simulink model "cemilModel"  (R2020b)
settings: Solver=VariableStepAuto  StartTime=0.0  StopTime=10.0  RelTol=1e-3
settings Model: Creator=kuzub  LastModifiedBy=kuzub

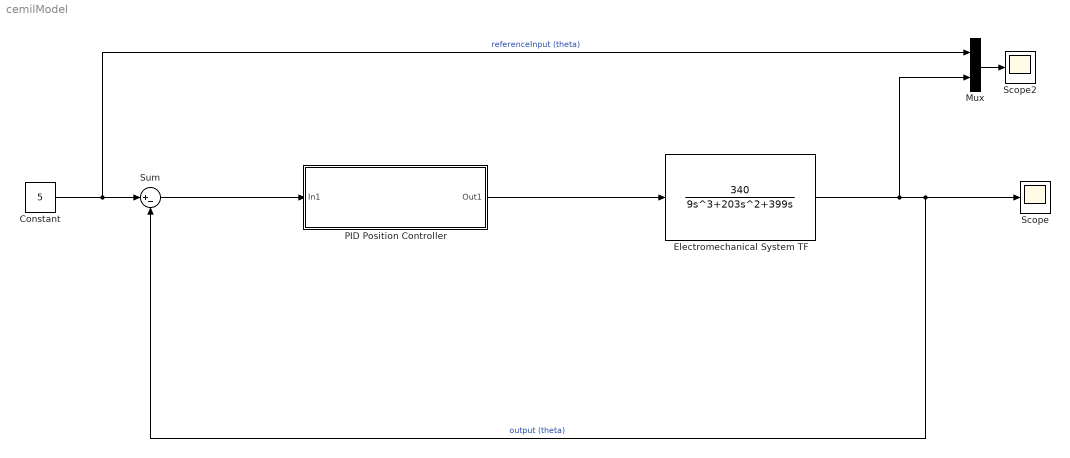
== system cemilModel ==
  Constant : Constant  Value=5
  Electromechanical System TF : TransferFcn  Numerator=[340]  Denominator=[9 203 399 0]
  Mux : Mux  Inputs=2
  PID Position Controller : Subsystem
  Scope : Scope
  Scope2 : Scope
  Sum : Sum  Inputs=|+-
  wires:
  Constant/1 -> Mux/1, Sum/1  "referenceInput (theta)"
  Electromechanical System TF/1 -> Mux/2, Scope/1, Sum/2  "output (theta)"
  Sum/1 -> PID Position Controller/1(In1)
  PID Position Controller/1(Out1) -> Electromechanical System TF/1
  Mux/1 -> Scope2/1

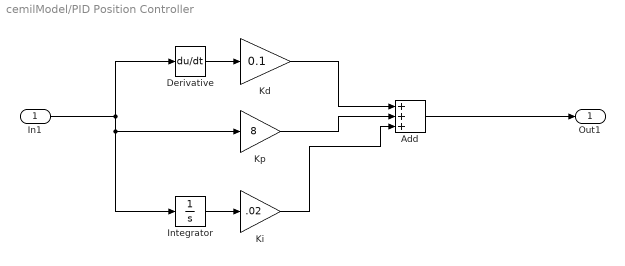
== system cemilModel/PID Position Controller ==
  In1 : Inport
  Add : Sum  Inputs=+++
  Derivative : Derivative
  Integrator : Integrator
  Kd : Gain  Gain=0.1
  Ki : Gain  Gain=.02
  Kp : Gain  Gain=8
  Out1 : Outport
  wires:
  Kd/1 -> Add/1
  In1/1 -> Derivative/1, Integrator/1, Kp/1
  Add/1 -> Out1/1
  Integrator/1 -> Ki/1
  Ki/1 -> Add/3
  Kp/1 -> Add/2
  Derivative/1 -> Kd/1
